simulink library "alfa_window_out"  (R2013b)
settings: Solver=ode45  StartTime=0.0  StopTime=10.0  RelTol=1e-3
libraries: carnot x2
settings Model: Creator=lena.frank  LastModifiedBy=drhf

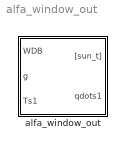
== system alfa_window_out ==
  alfa_window_out : Subsystem  mask(ALFA){pos=0, absorption_out=0.01, emission_out=0.87, frame=0.1}
      mask prompts: pos "Azimut of the surface (South = 0; East = -90)"; absorption_out "Solar absorption of the glass (0...1)"; emission_out "Longwave emissivity (0...1)"; frame "Share of the frame on the surface (0..1)"
      mask help:
      | Convective and radiative heat transfer at the OUTDOOR SURFACE OF A VERTICAL WINDOW.
      | Azimut can be a scalar or a vector with [inclination azimut rotation].
      | [W*] : modified weather data, adapted to height over ground,
      | Ts : temperature of outdoor window surface, °C,
      | qdots : specific heat flow into window construction, W/m^2,
      | [sun_t] : sun data (incidence angle, direct and diffuse radiation
      |                  at tilted window surface).
      mask init:
      | if length(pos) == 1
      |     pos = [90  pos 0]; % pos is [inclination azimut rotation]
      | end

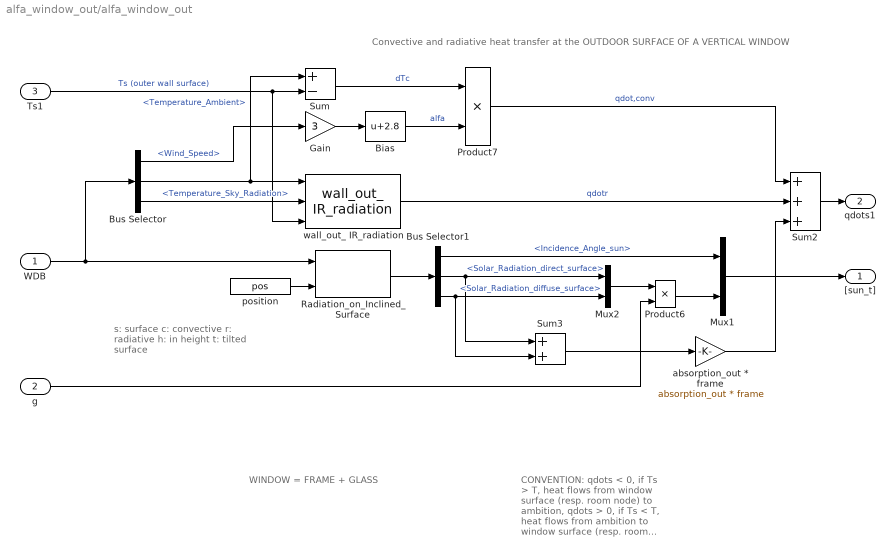
== system alfa_window_out/alfa_window_out ==
  note: WINDOW = FRAME + GLASS
  note: Convective and radiative heat transfer at the OUTDOOR SURFACE OF A VERTICAL WINDOW
  note: s: surface
      | c: convective
      | r: radiative
      | h: in height
      | t: tilted surface
  note: CONVENTION:
      | qdots < 0, if Ts > T, heat flows from window surface (resp. room node) to ambition,
      | qdots > 0, if Ts < T, heat flows from ambition to window surface (resp. room node).
  WDB : Inport
  g : Inport  Port=2
  Ts1 : Inport  Port=3
  Bias : Bias  Bias=2.8
  Bus Selector : BusSelector  OutputSignals=Wind_Speed,Temperature_Ambient,Temperature_Sky_Radiation
  Bus Selector1 : BusSelector  OutputSignals=Incidence_Angle_sun,Solar_Radiation_direct_surface,Solar_Radiation_diffuse_surface
  Gain : Gain  Gain=3
  Mux1 : Mux  Inputs=2
  Mux2 : Mux  Inputs=2
  Product6 : Product  SaturateOnIntegerOverflow=on  InputSameDT=on  OutDataTypeStr=Inherit: Same as first input
  Product7 : Product  SaturateOnIntegerOverflow=on  InputSameDT=on  OutDataTypeStr=Inherit: Same as first input
  Radiation_on_Inclined_Surface : carnot/Weather/Radiation_on_Inclined_Surface  sky=Perez 1990  reflect=0.2
  Sum : Sum  Inputs=+-  SaturateOnIntegerOverflow=on  InputSameDT=on  OutDataTypeStr=Inherit: Same as first input
  Sum2 : Sum  Inputs=+++  SaturateOnIntegerOverflow=on  InputSameDT=on  OutDataTypeStr=Inherit: Same as first input
  Sum3 : Sum  SaturateOnIntegerOverflow=on  InputSameDT=on  OutDataTypeStr=Inherit: Same as first input
  absorption_out * frame : Gain  Gain=absorption_out * frame  SaturateOnIntegerOverflow=on  OutDataTypeStr=Inherit: Same as input  ParamDataTypeStr=Inherit: Same as input
  position : Constant  Value=pos
  wall_out_ IR_radiation : carnot/Load/Houses/heat_transfer/wall_out_ IR_radiation
  "[sun_t]" : Outport
  qdots1 : Outport  Port=2
  wires:
  Radiation_on_Inclined_Surface/1 -> Bus Selector1/1
  position/1 -> Radiation_on_Inclined_Surface/2
  Product7/1 -> Sum2/1  "qdot,conv"
  Bias/1 -> Product7/2  "alfa"
  wall_out_ IR_radiation/1 -> Sum2/2  "qdotr"
  Ts1/1 -> Sum/2, wall_out_ IR_radiation/3  "Ts (outer wall surface)"
  Mux1/1 -> "[sun_t]"/1
  Bus Selector1/2 -> Mux2/1, Sum3/1  "<Solar_Radiation_direct_surface>"
  absorption_out * frame/1 -> Sum2/3
  g/1 -> Product6/2
  Sum2/1 -> qdots1/1
  Sum3/1 -> absorption_out * frame/1
  Bus Selector1/1 -> Mux1/1  "<Incidence_Angle_sun>"
  WDB/1 -> Radiation_on_Inclined_Surface/1, Bus Selector/1
  Sum/1 -> Product7/1  "dTc"
  Product6/1 -> Mux1/2
  Mux2/1 -> Product6/1
  Bus Selector1/3 -> Mux2/2, Sum3/2  "<Solar_Radiation_diffuse_surface>"
  Bus Selector/2 -> wall_out_ IR_radiation/1, Sum/1  "<Temperature_Ambient>"
  Bus Selector/3 -> wall_out_ IR_radiation/2  "<Temperature_Sky_Radiation>"
  Bus Selector/1 -> Gain/1  "<Wind_Speed>"
  Gain/1 -> Bias/1
